simulink model "TwoMassID_ref"  (R2022b)
settings: Solver=FixedStepDiscrete  StartTime=0.0  StopTime=160  FixedStep=0.000005  RelTol=1e-3  EnableMultiTasking=on
libraries: dspspect3 x1
settings Model: RequirementInfo={} %GIDa_fe9045fd_0412_4b6e_8206_617cc20e6fde  FPTRunName=Active  Creator=ts  LastModifiedBy=valen
settings SolverCC: AlgebraicLoopSolver=TrustRegion  PositivePriorityOrder=on  AutoInsertRateTranBlk=on
settings DataIOCC: SaveOutput=off  SignalLogging=off  DSMLogging=off  SaveTime=off
settings OptimizationCC: DefaultParameterBehavior=Inlined  UseDivisionForNetSlopeComputation=on  GainParamInheritBuiltInType=on  UseFloatMulNetSlope=on  DefaultUnderspecifiedDataType=single  UseSpecifiedMinMax=on  InlineInvariantSignals=on  PassReuseOutputArgsAs=Individual arguments  ZeroExternalMemoryAtStartup=off  ZeroInternalMemoryAtStartup=off  NoFixptDivByZeroProtection=on  EfficientFloat2IntCast=on  LifeSpan=1  MaxStackSize=64  OptimizeBlockOrder=speed  DifferentSizesBufferReuse=on  EfficientTunableParamExpr=on
settings DebuggingCC: UnconnectedInputMsg=warning  UnconnectedOutputMsg=warning  UnconnectedLineMsg=warning  BusObjectLabelMismatch=error  AllowSymbolicDim=off  SFUnexpectedBacktrackingDiag=warning  SFNoUnconditionalDefaultTransitionDiag=warning  SFExecutionAtInitializationDiag=none  SFMachineParentedDataDiag=warning  ArithmeticOperatorsInVariantConditions=warning
settings HardwareCC: ProdBitPerPointer=32  ProdBitPerSizeT=32  ProdBitPerPtrDiffT=32  ProdLargestAtomicInteger=Long  ProdLargestAtomicFloat=Double  ProdWordSize=32  ProdLongLongMode=on  ProdHWDeviceType=ARM Compatible->ARM Cortex-R  HardwareBoardFeatureSet=SoCBlockset
settings ModelReferenceCC: EnableRefExpFcnMdlSchedulingChecks=on
settings SFSimCC: SimGenImportedTypeDefs=on  MATLABDynamicMemAlloc=off
settings RTWCC: Description=Embedded Coder  SystemTargetFile=ert.tlc  GenCodeOnly=on  TemplateMakefile=ert_default_tmf  GenerateReport=on  BuildConfiguration=Faster Runs  IncludeHyperlinkInReport=on  LaunchReport=on  GenerateTraceInfo=on  GenerateTraceReport=on  GenerateTraceReportSl=on  GenerateTraceReportSf=on  GenerateTraceReportEml=on  GenerateCodeMetricsReport=on  CheckMdlBeforeBuild=Warning  DLArmComputeVersion=19.05
settings CodeAppCC: ForceParamTrailComments=on  IgnoreCustomStorageClasses=off  OperatorAnnotations=on  SimulinkDataObjDesc=on  SFDataObjDesc=on  MATLABFcnDesc=on  CustomSymbolStrGlobalVar=rt$M$R$N  CustomSymbolStrType=$N$M$R_t  CustomSymbolStrFcn=$N$M$F  CustomSymbolStrMacro=$N$M  InsertBlockDesc=on  StateflowObjectComments=on  MATLABSourceComments=on  EnableCustomComments=on  ReqsInCode=on
settings ERTTargetCC: TargetLangStandard=C99 (ISO)  CodeReplacementLibrary=GNU C99 extensions  UtilityFuncGeneration=Shared location  MultiwordLength=2048  IncludeMdlTerminateFcn=off  CombineSignalStateStructs=on  SuppressErrorStatus=on  IncludeFileDelimiter=UseQuote  SupportAbsoluteTime=off  CodeInterfacePackaging=Reusable function  RemoveResetFunc=off  InlinedParameterPlacement=NonHierarchical  MultiInstanceErrorCode=Warning  RootIOFormat=Part of model data structure  ERTCustomFileTemplate=example_file_process.tlc  GlobalDataDefinition=InSourceFile  GlobalDataReference=InSourceFile  ERTFilePackagingFormat=CompactWithDataFile  SuppressUnreachableDefaultCases=off
settings ConfigComp: CovScope=ReferencedModels  CovSaveName=covdata_rollAP  CovMetricSettings=dcmtrwe  CovHTMLOptions=-sRT=1 -aTS=1 -bRG=1 -bTC=1 -hTR=1 -nFC=0 -scm=1 -bcm=1 -xEv=0  CovSaveCumulativeToWorkspaceVar=on  CovSaveSingleToWorkspaceVar=on  CovCumulativeVarName=covCumulativeData_rollAP  CovReportOnPause=off  CovExternalEMLEnable=off  CovSFcnEnable=off

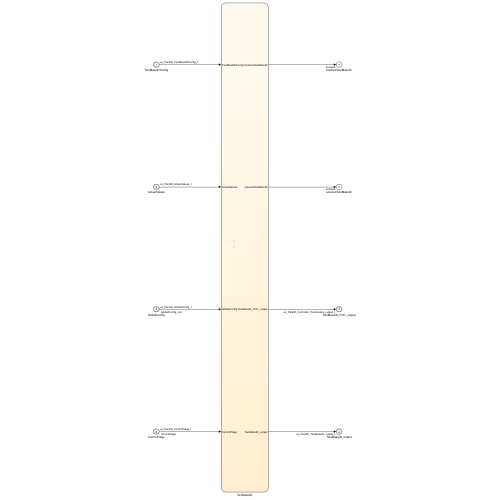
[thumbnail: Simulink's stored preview of the top-level diagram]
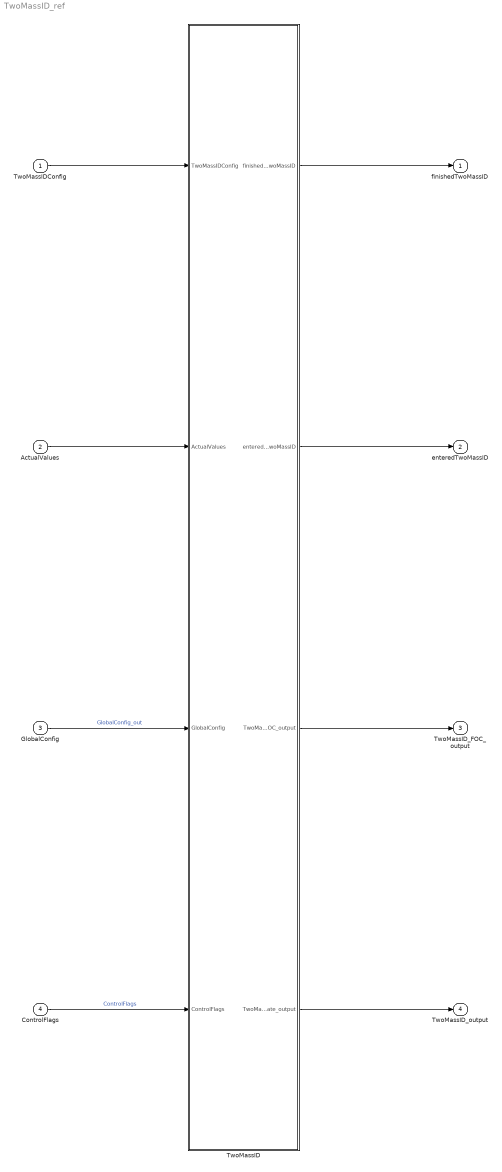
== system TwoMassID_ref ==
  TwoMassIDConfig : Inport  OutDataTypeStr=Bus: uz_ParaID_TwoMassIDConfig_t  PortDimensions=1  SampleTime=[5.0000000000000002e-05,0]  BusOutputAsStruct=on
  ActualValues : Inport  Port=2  OutDataTypeStr=Bus: uz_ParaID_ActualValues_t  PortDimensions=1  SampleTime=[5.0000000000000002e-05,0]  BusOutputAsStruct=on
  GlobalConfig : Inport  Port=3  OutDataTypeStr=Bus: uz_ParaID_GlobalConfig_t  PortDimensions=1  SampleTime=[5.0000000000000002e-05,0]  BusOutputAsStruct=on
  ControlFlags : Inport  Port=4  OutDataTypeStr=Bus: uz_ParaID_ControlFlags_t  PortDimensions=1  SampleTime=[5.0000000000000002e-05,0]  BusOutputAsStruct=on
  TwoMassID : Stateflow chart  TreatAsAtomicUnit=on
  finishedTwoMassID : Outport  OutDataTypeStr=boolean  PortDimensions=1  SampleTime=[5.0000000000000002e-05,0]
  enteredTwoMassID : Outport  Port=2  OutDataTypeStr=boolean  PortDimensions=1  SampleTime=[5.0000000000000002e-05,0]
  TwoMassID_FOC_output : Outport  Port=3  OutDataTypeStr=Bus: uz_ParaID_Controller_Parameters_output_t  PortDimensions=1  SampleTime=[5.0000000000000002e-05,0]  BusOutputAsStruct=on
  TwoMassID_output : Outport  Port=4  OutDataTypeStr=Bus: uz_ParaID_TwoMassID_output_t  PortDimensions=1  SampleTime=[5.0000000000000002e-05,0]  BusOutputAsStruct=on
  wires:
  TwoMassIDConfig/1 -> TwoMassID/1(TwoMassIDConfig)
  ActualValues/1 -> TwoMassID/2(ActualValues)
  GlobalConfig/1 -> TwoMassID/3(GlobalConfig)  "GlobalConfig_out"
  ControlFlags/1 -> TwoMassID/4(ControlFlags)  "ControlFlags"
  TwoMassID/1(finishedTwoMassID) -> finishedTwoMassID/1
  TwoMassID/2(enteredTwoMassID) -> enteredTwoMassID/1
  TwoMassID/3(TwoMassID_FOC_output) -> TwoMassID_FOC_output/1
  TwoMassID/4(TwoMassID_state_output) -> TwoMassID_output/1

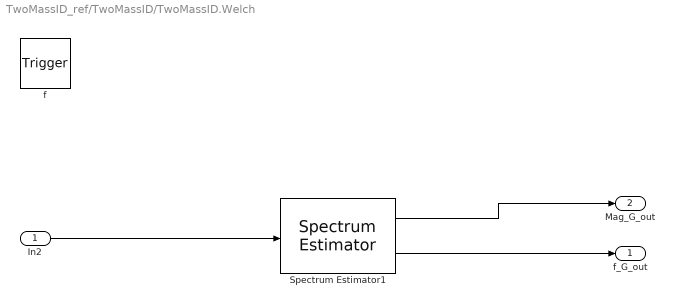
== system TwoMassID_ref/TwoMassID/TwoMassID.Welch ==
  In2 : Inport  OutDataTypeStr=single  Unit=Nm  PortDimensions=2046
  f : TriggerPort  TriggerType=function-call  VariantControl=(inherit)
      settings: CopyFcn=Stateflow.SLINSF.SimulinkMan.removeBlockPreDeleteFcn  PreDeleteFcn=Stateflow.SLINSF.SimulinkMan.unsafePredeleteFcn
  Spectrum Estimator1 : dspspect3/Spectrum Estimator  Method=Welch  NumTapsPerBand=12  SpectrumType=Power density  FrequencyResolutionMethod=Window length  FilterBankResolutionMethod=Auto  RBW=1  WindowLength=1024  FrequencyBandsSource=Same as input frame size  FrequencyBands=1024  FFTLengthSource=Property  FFTLength=2046  InheritSampleRate=off  SampleRate=1000  Window=Hann  SidelobeAttenuation=60  AveragingMethod=Running  SpectralAverages=1  ForgettingFactorPort=off  ForgettingFactor=0.9  Overlap=0  ReferenceLoad=1  FrequencyRange=One-sided  PowerUnits=dBm  OutputMaxHoldSpectrum=off  OutputMinHoldSpectrum=off  OutputFrequencyVector=on  OutputRBW=off  SimulateUsing=Code generation
  f_G_out : Outport  PortDimensions=1024  VectorParamsAs1DForOutWhenUnconnected=off
  Mag_G_out : Outport  Port=2  PortDimensions=1024  VectorParamsAs1DForOutWhenUnconnected=off
  wires:
  In2/1 -> Spectrum Estimator1/1
  Spectrum Estimator1/1 -> Mag_G_out/1
  Spectrum Estimator1/2 -> f_G_out/1

== stateflow chart TwoMassID_ref/TwoMassID ==
  settings: updateMethod=DISCRETE  sampleTime=1/d_f_states
  note: Two Mass System - identification
  state TwoMassID
    entry:
    initParams;
    enteredTwoMassID=boolean(1);
    TwoMassID_FOC_output.activeState=uint16(200);
    TwoMassID_FOC_output.enableFOC_speed=boolean(1);
    TwoMassID_FOC_output.resetIntegrator=boolean(1);
    during:
    state [f_G_out,Mag_G_out] = Welch(In2) [function]
    state TMS_Speed_State
      entry:
      TwoMassID_FOC_output.activeState = uint16(210);
      prbs_array(1:2047,1)=single(zeros(2047,1));
      counter=uint32(0);
      nextstate=uint32(0);
      mean_count=uint32(1);
      prbs_count=uint32(1);
      prbs_array(1:2047,1)=(single(PN)-0.5)*2*TwoMassIDConfig.ScaleTorquePRBS;
      TwoMassID_FOC_output.n_ref_FOC=single(0);
      TwoMassID_FOC_output.resetIntegrator=boolean(0);
      during:
      TwoMassID_FOC_output.n_ref_FOC=TwoMassIDConfig.n_ref_measurement;
      counter = counter +1;
      exit:
    state TMS_Noise_State
      entry:
      TwoMassID_FOC_output.activeState = uint16(220);
      TwoMassID_FOC_output.Ki_n_out=single(0.0);
      TwoMassID_FOC_output.Kp_n_out=single(0);
      omega_array(mean_count)=ActualValues.omega_m;
      iq_array(mean_count)=ActualValues.i_dq.q;
      during:
      counter=counter+1;
      mean_count=mean_count+1;
      if(mod(counter,uint32(0.001/GlobalConfig.sampleTimeISR))==0&&prbs_count<2047)
      prbs_count=prbs_count+1;
      end
      TwoMassID_state_output.PRBS_out=prbs_array(prbs_count);
      if(mean_count<1023)
      omega_array(mean_count)=ActualValues.omega_m;
      iq_array(mean_count)=ActualValues.i_dq.q;
      end
      if(mod(counter,uint32(0.001/GlobalConfig.sampleTimeISR))==0)
      nextstate=nextstate+1;
      J(nextstate,1)=sum(omega_array(1:1024))/single(mean_count);
      J(nextstate,2)=sum(iq_array(1:1024))/single(mean_count);
      mean_count=uint32(0);
      omega_array(1:1024)=zeros(1024,1);
      iq_array(1:1024)=zeros(1024,1);
      end
      exit:
      TwoMassID_state_output.PRBS_out=single(0);
      TwoMassID_FOC_output.n_ref_FOC=single(0);
      TwoMassID_FOC_output.Kp_n_out=GlobalConfig.Kp_n;
      TwoMassID_FOC_output.Ki_n_out=single(GlobalConfig.Ki_n);
    state TMS_calculate_state
      entry:
      TwoMassID_FOC_output.activeState = uint16(230);
      J(1:2048,2)=J(1:2048,2)*1.5*GlobalConfig.PMSM_config.polePairs*GlobalConfig.PMSM_config.Psi_PM_Vs;
      %omega Welch
      measArray1(1:1024)=zeros(1024,1);
      [measArray1(1:1024,1),measArray2(1:1024)] = Welch(J(1:2046,1));
      %torque Welch
      measArray2(1025:2048)=measArray2(1:1024);
      [measArray1(1:1024,1),measArray2(1:1024,1)] = Welch(J(1:2046,2));
      %G TMS
      measArray2(1:1024,1)=measArray2(1025:2048,1)-measArray2(1:1024,1);%Division in Time-Domain = Substraction in Frequ-Domain
      %TMS Noise
      LbMq=single(zeros(5,1));
      LbMq=Min_LbMq(measArray2(1:1024),measArray1(1:1024,1),TwoMassIDConfig.d_TMS_start,TwoMassIDConfig.f_min,TwoMassIDConfig.f_max,TwoMassIDConfig.UseLbMq);
      c_0_out=single(LbMq(1,1));
      TwoMassID_state_output.c_est_out=LbMq(2,1);
      TwoMassID_state_output.d_est_out=LbMq(3,1);
      TwoMassID_state_output.rotorInertia=LbMq(4,1);
      TwoMassID_state_output.LoadInertia=LbMq(5,1);
      TwoMassID_state_output.TrainInertia=TwoMassID_state_output.rotorInertia+TwoMassID_state_output.LoadInertia;
      c_max=single(TwoMassID_state_output.TrainInertia*4*3.14*3.14*500*500);
      counter=uint32(1);
      during:
      TwoMassID_FOC_output.resetIntegrator=boolean(1);
      counter = counter +1;
      exit:
      TwoMassID_FOC_output.resetIntegrator=boolean(0);
      TwoMassID_FOC_output.enableFOC_speed=boolean(0);
      finishedTwoMassID = boolean(1);
      enteredTwoMassID = boolean(0);
      reset_FOC_output;
    (default) -> TMS_Speed_State
    TMS_Speed_State -> TMS_Noise_State : [one_sec_transition_counter == counter]
    TMS_Noise_State -> TMS_calculate_state : [nextstate==2*1023]
  state Waiting
    entry:
    %wait for activation of
    %TwoMassID
    %donothing
  note: ---
  Waiting -> TwoMassID [order 1] : [ControlFlags.startTwoMassID==1 && GlobalConfig.Reset==0 && ....
      | GlobalConfig.ACCEPT==1]
  (default) -> Waiting
  Waiting -> Waiting [order 2] : [GlobalConfig.Reset==1]
      | {finishedTwoMassID=boolean(0);
      | enteredTwoMassID=boolean(0);
      | initParams;}
  TwoMassID -> Waiting : [GlobalConfig.Reset==1 || GlobalConfig.TwoMassID==0 || ....
      | GlobalConfig.enableParameterID==0]
      | {enteredTwoMassID=boolean(0);initParams;}
  TMS_calculate_state -> Waiting : [one_sec_transition_counter == counter]
  data: In2 function_input single size=2046; f_G_out function_output size=1024; Mag_G_out function_output size=1024; u function_output; uu function_output; Mag_G function_input; f_G function_input; d_start function_input; fmin function_input; fmax function_input; UseLevMar function_input; counter local uint32; Ustep local; mean_count local uint32; nextstate local; finishedTwoMassID output boolean; enteredTwoMassID output boolean; prbs_array local; prbs_count local; LbMq local; TwoMassIDConfig input Bus: uz_ParaID_TwoMassIDConfig_t; TwoMassID_FOC_output output Bus: uz_ParaID_Controller_Parameters_output_t; ActualValues input Bus: uz_ParaID_ActualValues_t; GlobalConfig input Bus: uz_ParaID_GlobalConfig_t; ControlFlags input Bus: uz_ParaID_ControlFlags_t; TwoMassID_state_output output Bus: uz_ParaID_TwoMassID_output_t; iq_array local; omega_array local; measArray2 local; measArray1 local; J local; c_0_out local; c_max local; one_sec_transition_counter local
  function u=PN:
    | function u=PN
    | pnSequence = comm.PNSequence('Polynomial',[11 9 0], ...
    |     'SamplesPerFrame',2047,'InitialConditions',[0 0 0 0 0 0 0 0 0 0 1]);
    |  u=pnSequence();
    |     end
  function uu=Min_LbMq(Mag_G,f_G,d_start,fmin,fmax,UseLevMar):
    | function uu=Min_LbMq(Mag_G,f_G,d_start,fmin,fmax,UseLevMar)
    |      
    |         Mag_G=Mag_G';
    |         index_min=uint16(0);
    |         index_max=uint16(0);
    |         lambda=single(1);
    |         nn_iters=uint16(50);
    |         G_est=single(0);
    |         G_est2=single(0);
    |         %coursor=single(zeros(200,13)); 
    |         Jac=single(zeros(1,2));
    |         Jac_0=single(zeros(1,2));
    |         y=single(zeros(2,1));
    |         H=single(zeros(2,2));
    |         H_0=single(zeros(2,2));
    |         pp=single(zeros(2,1));
    |         HyxHy=single(zeros(2,2));
    |         pxp=single(zeros(2,2));
    |         o=single(zeros(2,1));
    |         oxo=single(zeros(2,2));
    |         uuu=single(zeros(5,1));
    |         d1=single(0);
    |         ee=single(1);
    |         ee_lm=single(0);
    |         c_est=single(0);
    |         itt=uint16(0);
    |        
    | 
    |       %%%%%%%%%%%%%%%%%%%%%%%%%%%%%%%%%%%%%%%%%%%%%%%%%%%%%%%%%%%
    |       %                 FINDE Auswerte Bereich
    |       %%%%%%%%%%%%%%%%%%%%%%%%%%%%%%%%%%%%%%%%%%%%%%%%%%%%%%%%%%%
    |          for k=single(1):single(length(f_G))
    |       if(f_G(k)<fmin)
    |          index_min=uint16(k);
    |       end
    |       if(f_G(k)<fmax)
    |       index_max=uint16(k);
    |       end
    |          end
    |       
    |         
    |       %%%%%%%%%%%%%%%%%%%%%%%%%%%%%%%%%%%%%%%%%%%%%%%%%%%%%%%%%%%
    |       %                 FINDE MINIMUM
    |       %%%%%%%%%%%%%%%%%%%%%%%%%%%%%%%%%%%%%%%%%%%%%%%%%%%%%%%%%%%
    |         
    |       %finde Tigerfrequenz
    |       Tilgerwert=single(1000);
    |       Tilgerfrequenz=single(0);
    |       for k=single(index_min):single(index_max-1)
    |       if(Mag_G(k-1)>Mag_G(k)&&Mag_G(k)<Mag_G(k+1)&&Mag_G(k)<Tilgerwert)
    |           Tilgerwert=Mag_G(k);
    |           Tilgerfrequenz=f_G(k);
    |       end
    |       end
    |          %finde Resoanzfrequenz
    |       Resonanzwert=single(-1000);
    |       Resonanzfrequenz=single(0);
    |       for k=single(index_min):single(index_max-1)
    |       if(Mag_G(k-1)<Mag_G(k)&&Mag_G(k)>Mag_G(k+1)&&Mag_G(k)>Resonanzwert)
    |           Resonanzwert=Mag_G(k);
    |           Resonanzfrequenz=f_G(k);
    |       end
    |       end
    |       %Berechne JT
    |       JT=single(0);
    |       for k=single(index_min):single(index_min+10)
    |           JT=JT+1/(f_G(k+1)*2*pi*10^(Mag_G(k+1)/20));
    |           1/(f_G(k+1)*2*pi*10^(Mag_G(k+1)/20))
    |       end
    |       JT=JT/10;
    |       %Berechne JM, JL und c_start
    |       
    |       JL=JT*(1-(Tilgerfrequenz*Tilgerfrequenz)/(Resonanzfrequenz*Resonanzfrequenz))
    |       JM=JT-JL
    |         c_est_start=[JL*((Tilgerfrequenz*2*pi)^2),(JL*JM/(JL+JM))*(Resonanzfrequenz*2*pi)^2]
    |        
    |               
    |         %Fallunterscheidung Startwert nach Plausibliltaet
    |           
    |           if(c_est_start(1,1)>10&&c_est_start(1,2)<10)
    |         c_est=c_est_start(1,1);
    |           end
    |            if(c_est_start(1,1)<10&&c_est_start(1,2)>10)
    |         c_est=c_est_start(1,2);
    |            end
    |             if(c_est_start(1,1)<10&&c_est_start(1,2)<10)
    |         c_est=single(500);
    |             end
    |            if(c_est_start(1,1)>10&&c_est_start(1,2)>10)
    |         c_est=(c_est_start(1,2)+c_est_start(1,1))/2;
    |            end
    |         d_est=d_start;  
    |         uuu(1,1)=c_est;
    |        
    | if(UseLevMar==1)        
    | %Levenberg Marquardt Algorithm        
    |         c_lm=single(c_est);
    |         d_lm=single(d_est);
    |         updateJac=uint8(1);
    |         
    |     for itt=1:nn_iters
    |                 % itt
    |                 %coursor(itt,1)=c_est;
    |                  %coursor(itt,2)=d_est;
    |                  %coursor(itt,3)=updateJac;
    |                  
    |                  
    |         if updateJac == 1
    |             
    |            
    |             
    |         %Jacacobi-Matrix mit aktuellem Parametersatz berechnen
    |             fehler0=single(0);   
    |             Ustep=single(zeros(103,1));
    |              
    |                  
    |            for k=single(index_min):single(index_max)
    |         
    |            u=(c_est-JL*((f_G(k)*2*pi)^2)+d_est*(f_G(k)*2*pi)*i);
    |             v=(d_est*(-1)*((f_G(k)*2*pi)^2)*(JM+JL)+c_est*f_G(k)*2*pi*i*(JM+JL)-JM*JL*i*((f_G(k)*2*pi)^3));
    |             G_est= 20*log10(abs(u/v));
    |                 
    |             fehler0=fehler0+(Mag_G(1,k)-G_est)^2;
    |            end
    |             
    |            for m=single(1):single(50)
    |                
    |             fehlerc=single(0);
    |             c_est=c_est+0.1*(m-25.5);
    |               for k=single(index_min):single(index_max)
    |         
    |            u=(c_est-JL*((f_G(k)*2*pi)^2)+d_est*(f_G(k)*2*pi)*i);
    |             v=(d_est*(-1)*((f_G(k)*2*pi)^2)*(JM+JL)+c_est*f_G(k)*2*pi*i*(JM+JL)-JM*JL*i*((f_G(k)*2*pi)^3));
    |             G_est = 20*log10(abs(u/v));
    |             
    |             fehlerc=fehlerc+(Mag_G(1,k)-G_est)^2;
    |             end
    |              c_est=c_est-0.1*(m-25.5);   
    |              
    |                fehlerd=single(0);
    |                
    |             d_est=d_est+0.00001*(m-25.5);
    |              for k=single(index_min):single(index_max)
    |         
    |            u=(c_est-JL*((f_G(k)*2*pi)^2)+d_est*(f_G(k)*2*pi)*i);
    |             v=(d_est*(-1)*((f_G(k)*2*pi)^2)*(JM+JL)+c_est*f_G(k)*2*pi*i*(JM+JL)-JM*JL*i*((f_G(k)*2*pi)^3));
    |             G_est = 20*log10(abs(u/v));
    |             
    |             fehlerd=fehlerd+(Mag_G(1,k)-G_est)^2;
    |             end
    |              d_est=d_est-0.00001*(m-25.5);
    |              
    |          Ustep(m)=(fehlerc-fehler0)/(0.1*(m-25.5));
    |          Ustep(50+m)=(fehlerd-fehler0)/(0.00001*(m-25.5));
    |          
    |            end
    |            Ustep(1:50);
    |            Ustep(51:100);
    |         Jac(1)=mean(Ustep(1:50));
    |         Jac(2)=mean(Ustep(51:100));
    |          d1=fehler0;
    |          
    | %%Bestimmung Hessematrix          %%%%%%%%%%%%%%%%%%%%%%%%%%%%ana: Gauss Newton: H = Jac'*Jac;
    |             if itt==uint16(1)
    |                 ee = d1 %t(d1,d1)           % Fehlerquadrat berechnen
    |                 H=single(eye(2,2));
    |                     c_0=c_est;
    |                 d_0=d_est;
    |                 Jac_0=Jac;
    |                 H_0=H    ;
    |           end
    |             
    |          if itt>1
    |              itt
    |             % Gauss Newton: H = Jac'*Jac;
    |           H=Jac'*Jac;
    |               % Quasi Newton BFGS
    | %                 pc=c_est-c_0;
    | %                 pd=d_est-d_0;
    | %                 pp=[pc pd]';
    | %                 y=(Jac)'-Jac_0';
    | %                 Hy=H_0*y;
    | %                 yTHy=y'*Hy;
    | %                 pTy=pp'*y;
    | %                 o=pp/pTy-Hy/yTHy;
    | %                 pxp=pp*pp';
    | %                 HyxHy=Hy*Hy';
    | %                 oxo=o*o';
    | %                 B=pxp/pTy-HyxHy/yTHy+yTHy*oxo;
    | %                 H=B;
    | %                  c_0=c_est;
    | %                 d_0=d_est;
    | %                 Jac_0=Jac;
    | %                 H_0=H   ;     
    |                 
    |          end
    |  
    |        
    |             
    |             
    |         end
    |        % Daempfungsfaktor lambda auf Hesse-Matrix anwenden
    |         H(1,1) = H(1,1) + lambda; %Villwock: H=H+lambda*eye*H //Schroeder H=H+lambda*eye
    |         H(2,2)=H(2,2)+lambda;
    |              %coursor(itt,4)=Jac(1);
    |             %coursor(itt,5)=Jac(2);
    |          %coursor(itt,6)= det(H_0);
    |             
    |         %Neue Paramterschaetzung berechnen
    |         
    |         dp = single(-inv(H)*(Jac')*d1(:));%Schroeder:*d1(:)), Villwock ohne d1;
    |         %coursor(itt,7)=dp(1);
    |         %coursor(itt,8)=dp(2);
    |       
    |         if(c_est+real(dp(1))>0)
    |         c_lm =c_est +real(dp(1))
    |         else c_lm=single(0.1);
    |         end
    |         if(c_lm>10000)
    |             c_lm=single(10000);
    |         end
    |         if(d_est+real(dp(2))>0)
    |         d_lm = d_est  + real(dp(2))
    |         else
    |             d_lm=single(0.000001);
    |         end
    |         
    |         if(d_lm>10)
    |             d_lm=single(10);
    |         end
    |         ee_lm=single(0);
    |         d2=single(0);
    |        % Modellfunktion mit neuem Parametersatz berechnen
    |         for k=single(index_min):single(index_max)
    |         G_est2= 20*log10(abs((c_lm-JL*((f_G(k)*2*pi)^2)+d_lm*(f_G(k)*2*pi)*i)/(d_lm*(-1)*((f_G(k)*2*pi)^2)*(JM+JL)+c_lm*f_G(k)*2*pi*i*(JM+JL)-JM*JL*i*((f_G(k)*2*pi)^3))));
    |         if(d2<single(1*10^38))
    |         d2 = d2 +abs(Mag_G(1,k) - G_est2)^2;
    |         else
    |         d2=single(0);
    |         ee_lm=single(1*10^38);
    |         end        
    |         end
    |         
    |         %Auswertefehler setzen
    |         if(ee_lm==0)
    |         ee_lm = d2        
    |         end
    |         %coursor(itt,9)=c_lm;
    |         %coursor(itt,10)=d_lm;
    |         %coursor(itt,11)=d1;%e
    |         %coursor(itt,12)=d2;%e_lm
    |         %coursor(itt,13)=lambda;
    |         
    |        % Fallunterscheidung ob Fehler groesser oder kleiner geworden ist
    |         if ee_lm <= ee
    |             lambda = lambda/2;
    |             c_est = c_lm
    |            d_est = d_lm
    |            ee = ee_lm;
    |             updateJac = uint8(1);
    |             if(abs(dp(1))< single(0.0001) && abs(dp(2))< single(0.0000001))
    |                 dp(1)
    |                 dp(2)
    |                 break
    |             end
    |          
    |             
    |         end
    |              
    |         if ee_lm > ee
    |             updateJac = uint8(0);
    |             lambda = lambda*10;
    |         end
    |    
    | 
    | 
    |  %Pruefen ob Abbruchbedingung erreicht
    |         if ee<=500
    |             ee
    |            break
    |         end
    | 
    |     end
    | end
    | 
    | if(UseLevMar==0)
    | %Schaetze Daempfung ueber Amplitudengangwerte an f_res und f_Til
    | 
    | d_til =  abs((JL*(Tilgerfrequenz*2*pi)^2 - c_est+(c_est*(JM+JL)-JM*JL*(Tilgerfrequenz*2*pi)^2)*Tilgerfrequenz*2*pi*10^(Tilgerwert/20)*i)    /   ((10^(Tilgerwert/20))*(Tilgerfrequenz*2*pi)^2 *(JM+JL)  + Tilgerfrequenz*2*pi*i     ))
    | d_res =  abs((JL*(Resonanzfrequenz*2*pi)^2 - c_est+(c_est*(JM+JL)-JM*JL*(Resonanzfrequenz*2*pi)^2)*Resonanzfrequenz*2*pi*10^(Resonanzwert/20)*i)    /   ((10^(Resonanzwert/20))*(Resonanzfrequenz*2*pi)^2 *(JM+JL)  + Resonanzfrequenz*2*pi*i   )  )
    | d_est=single((d_res+d_til)/2);
    | 
    | 
    | end
    |         
    | 
    | uuu(2,1)=c_est;
    | uuu(3,1)=d_est;
    | uuu(4,1)=JM;
    | uuu(5,1)=JL;
    | %uuu(4:203,1:13)=%coursor;
    |         uu=uuu;
  function initParams:
    | function initParams
    | 
    | %This is used instead of "after(1.0,sec) to ensure the same transition time
    | %independelty of the sampletime in the c-code
    | one_sec_transition_counter = uint32(1/GlobalConfig.sampleTimeISR);
    | % initialize variables
    | measArray1			= single(zeros(1024,1));
    | J 					= single(zeros(2048,2));
    | prbs_array        	= single(zeros(2048,1));
    | measArray2 			= single(zeros(2048,1));
    | iq_array            = single(zeros(1024,1));
    | omega_array         = single(zeros(1024,1));
    | %Outputs
    | TwoMassID_FOC_output.n_ref_FOC      	= single(0.0);
    | TwoMassID_FOC_output.M_ref_FOC      	= single(0.0);
    | TwoMassID_FOC_output.i_dq_ref.d         = single(0.0);
    | TwoMassID_FOC_output.i_dq_ref.q         = single(0.0);
    | TwoMassID_FOC_output.i_dq_ref.zero      = single(0.0);
    | TwoMassID_FOC_output.enableFOC_speed	= boolean(0);
    | TwoMassID_FOC_output.enableFOC_current	= boolean(0);
    | TwoMassID_FOC_output.enableFOC_torque   = boolean(0);
    | TwoMassID_FOC_output.resetIntegrator 	= boolean(0);
    | finishedTwoMassID   = boolean(0);
    | TwoMassID_FOC_output.Kp_id_out          = single(GlobalConfig.Kp_id);
    | TwoMassID_FOC_output.Kp_iq_out          = single(GlobalConfig.Kp_iq);
    | TwoMassID_FOC_output.Kp_n_out           = single(GlobalConfig.Kp_n);
    | TwoMassID_FOC_output.Ki_id_out          = single(GlobalConfig.Ki_id);
    | TwoMassID_FOC_output.Ki_iq_out      	= single(GlobalConfig.Ki_iq);
    | TwoMassID_FOC_output.Ki_n_out           = single(GlobalConfig.Ki_n);
    | TwoMassID_state_output.c_est_out              = single(0.0); 
    | TwoMassID_state_output.d_est_out              = single(0.0);
    | TwoMassID_FOC_output.activeState        = uint16(0);
    | TwoMassID_state_output.LoadInertia            = single(0.0);
    | TwoMassID_state_output.TrainInertia           = single(0.0);
    | TwoMassID_state_output.rotorInertia           = single(0.0);
    | TwoMassID_state_output.PRBS_out               = single(0.0);
    | end
  function reset_FOC_output:
    | function reset_FOC_output
    | 
    | %Outputs
    | TwoMassID_FOC_output.n_ref_FOC      	= single(0.0);
    | TwoMassID_FOC_output.M_ref_FOC      	= single(0.0);
    | TwoMassID_FOC_output.i_dq_ref.d         = single(0.0);
    | TwoMassID_FOC_output.i_dq_ref.q         = single(0.0);
    | TwoMassID_FOC_output.i_dq_ref.zero      = single(0.0);
    | TwoMassID_FOC_output.enableFOC_speed	= boolean(0);
    | TwoMassID_FOC_output.enableFOC_current	= boolean(0);
    | TwoMassID_FOC_output.enableFOC_torque   = boolean(0);
    | TwoMassID_FOC_output.resetIntegrator 	= boolean(0);
    | TwoMassID_FOC_output.Kp_id_out          = single(GlobalConfig.Kp_id);
    | TwoMassID_FOC_output.Kp_iq_out          = single(GlobalConfig.Kp_iq);
    | TwoMassID_FOC_output.Kp_n_out           = single(GlobalConfig.Kp_n);
    | TwoMassID_FOC_output.Ki_id_out          = single(GlobalConfig.Ki_id);
    | TwoMassID_FOC_output.Ki_iq_out      	= single(GlobalConfig.Ki_iq);
    | TwoMassID_FOC_output.Ki_n_out           = single(GlobalConfig.Ki_n);
    | TwoMassID_FOC_output.activeState        = uint16(0);
    | 
    | end
